simulink library "hysteresisSwitch_ul"  (R2018b)
settings: Solver=VariableStepAuto  StartTime=0.0  StopTime=10.0  RelTol=1e-3
settings Model: Creator=mcobb  LastModifiedBy=mcobb

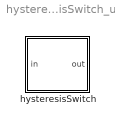
== system hysteresisSwitch_ul ==
  hysteresisSwitch : Stateflow chart  TreatAsAtomicUnit=on  mask{upperLim=0, lowerLim=0}
      mask prompts: upperLim "Upper Limit"; lowerLim "Lower Limit"

== stateflow chart hysteresisSwitch_ul/hysteresisSwitch ==
  state ON
  state OFF
  (default) -> OFF
  ON -> OFF : [in<lowerLim]{out=false;}
  OFF -> ON : [in>upperLim]{out=true;}
  data: in input; out output; upperLim parameter; lowerLim parameter
